simulink model "logic_expand_2_test"  (Simulink 9.0)
settings: Solver=FixedStepAuto  StartTime=0.0  StopTime=10.0  FixedStep=0.1  RelTol=1e-3  EnableMultiTasking=on
settings Model: SuppressorTable=22 serialization::archive 11 0 6 0 0 0 0 0  Creator=arnaud  LastModifiedBy=hbourbou
settings DataIOCC: LimitDataPoints=on  SaveFormat=Structure  SignalLoggingSaveFormat=ModelDataLogs
settings OptimizationCC: ExpressionDepthLimit=2147483647
settings DebuggingCC: SolverPrmCheckMsg=warning  FcnCallInpInsideContextMsg=warning  StateNameClashWarn=warning  StrictBusMsg=Warning
settings GRTTargetCC: CombineOutputUpdateFcns=off  GRTInterface=on

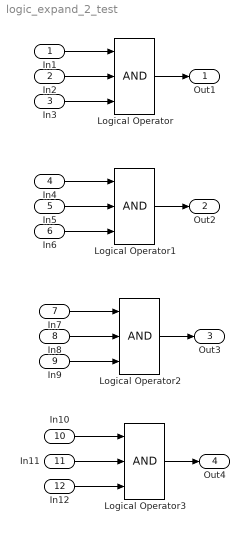
== system logic_expand_2_test ==
  In1 : Inport  PortDimensions=1
  In2 : Inport  Port=2  PortDimensions=[2 3]
  In3 : Inport  Port=3  PortDimensions=1
  In4 : Inport  Port=4  PortDimensions=[2 3]
  In5 : Inport  Port=5  PortDimensions=1
  In6 : Inport  Port=6  PortDimensions=[2 3]
  In7 : Inport  Port=7  PortDimensions=1
  In8 : Inport  Port=8  PortDimensions=1
  In9 : Inport  Port=9  PortDimensions=[2 3]
  In10 : Inport  Port=10  PortDimensions=[2 3]
  In11 : Inport  Port=11  PortDimensions=1
  In12 : Inport  Port=12  PortDimensions=1
  Logical Operator{,1..3} (4 alike) : Logic  Inputs=3  AllPortsSameDT=off  OutDataTypeStr=boolean
  Out1 : Outport
  Out2 : Outport  Port=2
  Out3 : Outport  Port=3
  Out4 : Outport  Port=4
  wires:
  In1/1 -> Logical Operator/1
  Logical Operator/1 -> Out1/1
  In2/1 -> Logical Operator/2
  In3/1 -> Logical Operator/3
  In4/1 -> Logical Operator1/1
  Logical Operator1/1 -> Out2/1
  In5/1 -> Logical Operator1/2
  In6/1 -> Logical Operator1/3
  In7/1 -> Logical Operator2/1
  Logical Operator2/1 -> Out3/1
  In8/1 -> Logical Operator2/2
  In9/1 -> Logical Operator2/3
  In10/1 -> Logical Operator3/1
  Logical Operator3/1 -> Out4/1
  In11/1 -> Logical Operator3/2
  In12/1 -> Logical Operator3/3
